simulink model "GTSim_RQ"  (Simulink 7.8)
settings: Solver=ode45  StartTime=0.0  StopTime=3000  RelTol=1e-3
undefined symbols (not defined in the file or in its folder): des_subsystemblock, des_subsysteminport, des_subsystemoutport, des_subsystemsupportblock, MARGIN
libraries: simeventsattributes2 x20, simeventssink1 x17, simeventsrouting1 x15, simeventsgenerators1 x12, simeventstiming1 x4, simeventsqueue1 x1, simeventstranslate1 x1, simeventsserver1 x1
settings Model: Creator=msemamit  LastModifiedBy=msemamit
settings DebuggingCC: FcnCallInpInsideContextMsg=Use local settings
settings SFSimCC: SimParseCustomCode=off
settings SimEventsCC: propDiagAttribOutput=1  propDiagFcnCallOutput=1  propDiagStatOutput=0

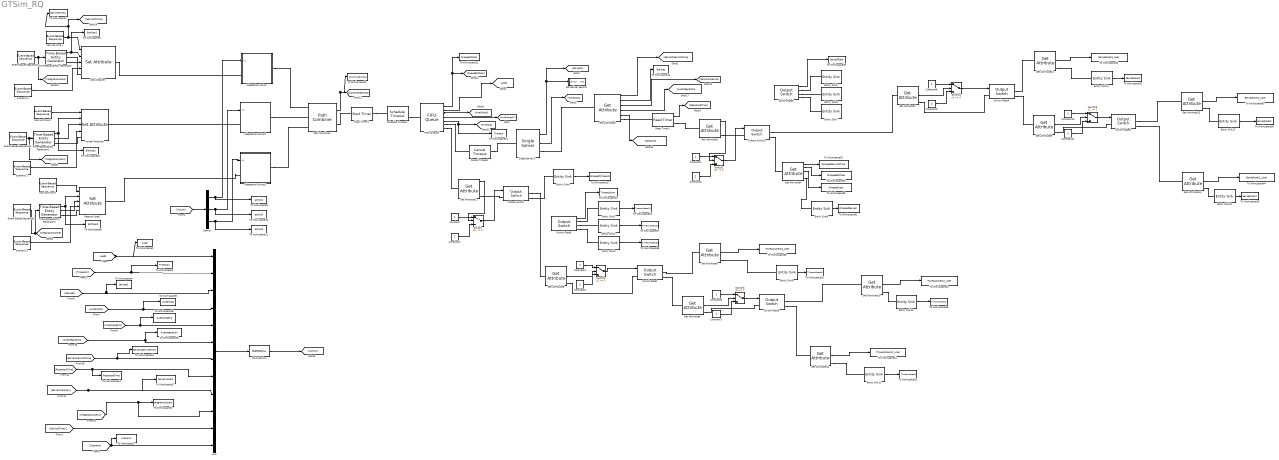
== system GTSim_RQ ==
  Adaptation Action : Subsystem
  Adaptation Action1 : Subsystem
  Adaptation Action2 : Subsystem
  Cancel Timeout : simeventstiming1/Cancel Timeout  Priority=0  TimeoutTag=TO1  TimeoutModeOption=Continue  TimeoutCancelledOption=Error  StatNumberDeparted=Off  StatTimeoutNumberDeparted=Off  StatResidualTimeout=Off  StatAverageResidualTimeout=Off
  Constant{,2,4,6,8,10} (6 alike) : Constant  OutDataTypeStr=double
  Constant{1,3,5,7,9,11} (6 alike) : Constant  Value=2  OutDataTypeStr=double
  Demux : Demux  Outputs=3
  DoS Attacker : simeventsattributes2/Set Attribute  Priority=1  AttributeFrom=Signal port|Signal port|Dialog|Signal port|Signal port  AttributeName=ServiceTime|Entities|User|AveIntegration|Scenario  AttributeTreatAsVector=1|1|1|1|1  AttributeValue=1|1|1|1|1  AttributeCreate=on  StatNumberDeparted=Off  EvaluatedAttributeValue={[];[];1;[];[]}
  Entity Sink{1..14} (14 alike) : simeventssink1/Entity Sink  Priority=1  AvailableForArrivals=on  StatNumberArrived=On
  Event-Based Sequence : simeventsgenerators1/Signal Generators/Event-Based Sequence  VectorOutputValues=user1  FormOutputOpt=Setting to infinity  IsProcessed=on  isConnected=1
  Event-Based Sequence1 : simeventsgenerators1/Signal Generators/Event-Based Sequence  VectorOutputValues=user2  FormOutputOpt=Setting to infinity  IsProcessed=on  isConnected=1
  Event-Based Sequence2 : simeventsgenerators1/Signal Generators/Event-Based Sequence  VectorOutputValues=user3  FormOutputOpt=Setting to infinity  IsProcessed=on  isConnected=1
  FIFO Queue7 : simeventsqueue1/FIFO Queue  Priority=1  Capacity=5000  EnableTOPort=on  StatNumberDeparted=On  StatNumberInBlock=On  StatPendingEntity=Off  StatAverageWait=On  StatAverageQueueLength=On  StatNumberTimedout=On
  Get Attribute{1,3..14} (13 alike) : simeventsattributes2/Get Attribute  Priority=1  AttributeName=ServiceTime|Entities|User|AveIntegration  AttributeMissing=Error|Error|Error|Error  AttributeDefaultValue=1|1|1|1  AttributeSendTiming=After entity departure|After entity departure|After entity departure|After entity departure  AttributeTreatAsVector=1|1|1|1  StatNumberDeparted=Off  EvaluatedDefaultAttributeValue={[];[];[];[]}
  Get Attribute2 : simeventsattributes2/Get Attribute  Priority=1  AttributeName=ServiceTime|Entities|User|AveIntegration|Scenario  AttributeMissing=Error|Error|Error|Error|Error  AttributeDefaultValue=1|1|1|1|1  AttributeSendTiming=After entity departure|After entity departure|After entity departure|After entity departure|After entity departure  AttributeTreatAsVector=1|1|1|1|1  StatNumberDeparted=Off  EvaluatedDefaultAttributeValue={[];[];[];[];[]}
  Insider Attacker : simeventsattributes2/Set Attribute  Priority=1  AttributeFrom=Signal port|Signal port|Dialog|Signal port|Signal port  AttributeName=ServiceTime|Entities|User|AveIntegration|Scenario  AttributeTreatAsVector=1|1|1|1|1  AttributeValue=1|1|2|1|1  AttributeCreate=on  StatNumberDeparted=Off  EvaluatedAttributeValue={[];[];2;[];[]}
  MATLAB Fcn : MATLABFcn  MATLABFcn=MARGIN(u)
  Mux : Mux  Inputs=12
  Output Switch : simeventsrouting1/Output Switch  Priority=1  NumberOutputPorts=2  SwitchingCriterion=From signal port p  InitialSeed=34567  AttributeName=Attribute1  InitialConditionsOpt=off  InitialConditions=1  EntityBufferOpt=on  SpecifyEventPriority=off  PriorityOutputSwitchSelectPort=4100  TimeoutPortOpt=off  StatNumberDeparted=On  StatNumberTimedOut=Off  StatPendingEntity=Off  StatLastDeparturePort=Off  EvaluatedNumPorts=2
  Output Switch1 : simeventsrouting1/Output Switch  Priority=1  NumberOutputPorts=2  SwitchingCriterion=From signal port p  InitialSeed=34567  AttributeName=Attribute1  InitialConditionsOpt=off  InitialConditions=1  EntityBufferOpt=on  SpecifyEventPriority=off  PriorityOutputSwitchSelectPort=4100  TimeoutPortOpt=off  StatNumberDeparted=On  StatNumberTimedOut=Off  StatPendingEntity=Off  StatLastDeparturePort=Off  EvaluatedNumPorts=2
  Path Combiner : simeventsrouting1/Path Combiner  Priority=1  NumberInputPorts=3  InputPortPrecedence=Round robin  InitialSeed=45675  SpecifyEventPriority=off  PriorityPathCombinerPortPrecedenceSelection=4100  StatNumberDeparted=On  StatLastArrivalPort=Off  EvaluatedNumPorts=3
  Read Timer1 : simeventstiming1/Read Timer  Priority=0  TimerTag=T2  TimerModeOption=Error  TimerStop=off  StatNumberDeparted=Off  StatTimerNumberDeparted=Off  StatTimeElapsed=On  StatAverageTimeElapsed=Off
  Regular User1 : simeventsattributes2/Set Attribute  Priority=1  AttributeFrom=Signal port|Signal port|Dialog|Signal port|Signal port  AttributeName=ServiceTime|Entities|User|AveIntegration|Scenario  AttributeTreatAsVector=1|1|1|1|1  AttributeValue=1|1|3|1|1  AttributeCreate=on  StatNumberDeparted=Off  EvaluatedAttributeValue={[];[];3;[];[]}
  Schedule Timeout : simeventstiming1/Schedule Timeout  Priority=0  TimeoutTag=TO1  TimeoutIntervalFrom=Dialog  TimeoutInterval=3000  AttributeName=TimeoutAttribute  PriorityTimeout=1700  TimeoutScheduledOption=Error  TimeoutNoDestination=Error  StatNumberDeparted=On
  Served per Second : Subsystem  LoadFcn=des_subsystemblock(gcb, 'load');  InitFcn=des_subsystemblock(gcb, 'init');  StartFcn=des_subsystemblock(gcb, 'start');  StopFcn=des_subsystemblock(gcb, 'stop');
      settings: CopyFcn=des_subsystemblock(gcb, 'copy');  DeleteFcn=des_subsystemblock(gcb, 'delete');  UndoDeleteFcn=des_subsystemblock(gcb, 'undodelete');  ModelCloseFcn=des_subsystemblock(gcb, 'modelclose');  PreSaveFcn=des_subsystemblock(gcb, 'presave');  NameChangeFcn=des_subsystemblock(gcb, 'namechange');  OpenFcn=des_subsystemblock(gcb, 'open');  ParentCloseFcn=des_subsystemblock(gcb, 'parentclose');  ErrorFcn=des_subsystemerror
      mask Type: Discrete Event Subsystem
      mask Help: helpview(simeventsbhelp);
  Single Server 1 : simeventsserver1/Single Server  Priority=1  ServiceTimeFrom=Attribute  ServiceTime=1  AttributeName=ServiceTime  PriorityServiceCompletion=500  PermitPreemption=off  SortingAttributeName=PriorityAttributeName  SortingDirection=Ascending  WriteToAttribute=off  ResidualAttributeName=ResidualServiceTime  CreateAttribute=on  EnableTOPort=off  StatNumberDeparted=On  StatNumberInBlock=Off  StatNumberPreempted=Off  StatPendingEntity=Off  StatAverageWait=Off  StatUtilization=Off  StatNumberTimedout=On
  Start Timer1 : simeventstiming1/Start Timer  Priority=0  TimerTag=T2  TimerStartedOption=Warn and continue  StatNumberDeparted=Off
  Switch : Switch  Criteria=u2 ~= 0  ZeroCross=off
  Switch Gate{1,3..4,6} (4 alike) : simeventsrouting1/Output Switch  Priority=1  NumberOutputPorts=2  SwitchingCriterion=From signal port p  InitialSeed=34567  AttributeName=User  InitialConditionsOpt=off  InitialConditions=1  EntityBufferOpt=on  SpecifyEventPriority=off  PriorityOutputSwitchSelectPort=4100  TimeoutPortOpt=off  StatNumberDeparted=On  StatNumberTimedOut=Off  StatPendingEntity=Off  StatLastDeparturePort=Off  EvaluatedNumPorts=2
  Switch Gate2 : simeventsrouting1/Output Switch  Priority=1  NumberOutputPorts=3  SwitchingCriterion=From attribute  InitialSeed=34567  AttributeName=User  InitialConditionsOpt=off  InitialConditions=1  EntityBufferOpt=off  SpecifyEventPriority=off  PriorityOutputSwitchSelectPort=4100  TimeoutPortOpt=off  StatNumberDeparted=On  StatNumberTimedOut=Off  StatPendingEntity=Off  StatLastDeparturePort=Off  EvaluatedNumPorts=3
  Switch Gate5 : simeventsrouting1/Output Switch  Priority=1  NumberOutputPorts=3  SwitchingCriterion=From attribute  InitialSeed=34567  AttributeName=User  InitialConditionsOpt=off  InitialConditions=1  EntityBufferOpt=off  SpecifyEventPriority=off  PriorityOutputSwitchSelectPort=4100  TimeoutPortOpt=off  StatNumberDeparted=On  StatNumberTimedOut=Off  StatPendingEntity=Off  StatLastDeparturePort=Off  EvaluatedNumPorts=3
  Switch1 : Switch  Criteria=u2 ~= 0  ZeroCross=off
  Switch2 : Switch  Threshold=3  ZeroCross=off
  Switch3 : Switch  Threshold=2  ZeroCross=off
  Switch4 : Switch  Threshold=3  RndMeth=Ceiling  ZeroCross=off
  Switch5 : Switch  Threshold=2  RndMeth=Ceiling  ZeroCross=off
  Time-Based Entity Generator : simeventsgenerators1/Entity Generators/Time-Based Entity Generator  Priority=1  GenerateEntitiesUpon=Intergeneration time from port t  Distribution=Constant  Minimum=50  Maximum=100  Mean=15  InitialSeed=12345  Period=5  PriorityEntityGeneration=300  GenerateEntityAtSimulationStart=on  ResponseWhenBlocked=Error  ResponseWhenUnblocked=Immediate restart  EntityType=Blank  StatNumberDeparted=On  StatPendingEntity=Off  StatAverageIntergenerationTime=On
  Time-Based Entity Generator1 : simeventsgenerators1/Entity Generators/Time-Based Entity Generator  Priority=1  GenerateEntitiesUpon=Intergeneration time from port t  Distribution=Constant  Minimum=10  Maximum=100  Mean=10  InitialSeed=12345  Period=50  PriorityEntityGeneration=300  GenerateEntityAtSimulationStart=on  ResponseWhenBlocked=Error  ResponseWhenUnblocked=Immediate restart  EntityType=Blank  StatNumberDeparted=On  StatPendingEntity=Off  StatAverageIntergenerationTime=On
  Time-Based Entity Generator2 : simeventsgenerators1/Entity Generators/Time-Based Entity Generator  Priority=1  GenerateEntitiesUpon=Intergeneration time from port t  Distribution=Constant  Minimum=10  Maximum=100  Mean=10  InitialSeed=12345  Period=50  PriorityEntityGeneration=300  GenerateEntityAtSimulationStart=on  ResponseWhenBlocked=Error  ResponseWhenUnblocked=Immediate restart  EntityType=Blank  StatNumberDeparted=On  StatPendingEntity=Off  StatAverageIntergenerationTime=On
  To Workspace1 : ToWorkspace  VariableName=ServiceTime1  SampleTime=-1  SaveFormat=Array
  To Workspace10 : ToWorkspace  VariableName=action2  SampleTime=-1  SaveFormat=Array
  To Workspace11 : ToWorkspace  VariableName=action3  SampleTime=-1  SaveFormat=Array
  To Workspace12 : ToWorkspace  VariableName=ResponseTime  SampleTime=-1  SaveFormat=Array
  To Workspace13 : ToWorkspace  VariableName=Timeout  SampleTime=-1  SaveFormat=Array
  To Workspace14 : ToWorkspace  VariableName=Entities  SampleTime=-1  SaveFormat=Array
  To Workspace15 : ToWorkspace  VariableName=Server1ServiceTime  SampleTime=-1  SaveFormat=Array
  To Workspace16 : ToWorkspace  VariableName=AveQLength1  SampleTime=-1  SaveFormat=Array
  To Workspace17 : ToWorkspace  VariableName=Server1Users  SampleTime=-1  SaveFormat=Array
  To Workspace18 : ToWorkspace  VariableName=AveIntegration  SampleTime=-1  SaveFormat=Array
  To Workspace19 : ToWorkspace  VariableName=Entities2  SampleTime=-1  SaveFormat=Array
  To Workspace2 : ToWorkspace  VariableName=Load  SampleTime=-1  SaveFormat=Array
  To Workspace20 : ToWorkspace  VariableName=IntegrationUser1  SampleTime=-1  SaveFormat=Array
  To Workspace21 : ToWorkspace  VariableName=QueueEntities  SampleTime=-1  SaveFormat=Array
  To Workspace22 : ToWorkspace  VariableName=CombinerEntities  SampleTime=-1  SaveFormat=Array
  To Workspace23 : ToWorkspace  VariableName=TimeoutUsers11  SampleTime=-1  SaveFormat=Array
  To Workspace24 : ToWorkspace  VariableName=TimeoutNum  SampleTime=-1  SaveFormat=Array
  To Workspace25 : ToWorkspace  VariableName=TimeoutUsers1  SampleTime=-1  SaveFormat=Array
  To Workspace26 : ToWorkspace  VariableName=TimeoutUsers3  SampleTime=-1  SaveFormat=Array
  To Workspace27 : ToWorkspace  VariableName=DroppedTimeouts  SampleTime=-1  SaveFormat=Array
  To Workspace28 : ToWorkspace  VariableName=ServedUser1  SampleTime=-1  SaveFormat=Array
  To Workspace29 : ToWorkspace  VariableName=ServedTotal  SampleTime=-1  SaveFormat=Array
  To Workspace3 : ToWorkspace  VariableName=Timeout1  SampleTime=-1  SaveFormat=Array
  To Workspace30 : ToWorkspace  VariableName=ServedUser2  SampleTime=-1  SaveFormat=Array
  To Workspace31 : ToWorkspace  VariableName=ServedUser3  SampleTime=-1  SaveFormat=Array
  To Workspace32 : ToWorkspace  VariableName=DroppedServed  SampleTime=-1  SaveFormat=Array
  To Workspace33 : ToWorkspace  VariableName=DroppedServiceTime  SampleTime=-1  SaveFormat=Array
  To Workspace34 : ToWorkspace  VariableName=DroppedEntities  SampleTime=-1  SaveFormat=Array
  To Workspace35 : ToWorkspace  VariableName=DroppedUser  SampleTime=-1  SaveFormat=Array
  To Workspace36 : ToWorkspace  VariableName=TimeoutUsers2  SampleTime=-1  SaveFormat=Array
  To Workspace37 : ToWorkspace  VariableName=TimeoutUsers22  SampleTime=-1  SaveFormat=Array
  To Workspace38 : ToWorkspace  VariableName=TimeoutUsers33  SampleTime=-1  SaveFormat=Array
  To Workspace39 : ToWorkspace  VariableName=TimeoutUsers3_User  SampleTime=-1  SaveFormat=Array
  To Workspace4 : ToWorkspace  VariableName=Served1  SampleTime=-1  SaveFormat=Array
  To Workspace40 : ToWorkspace  VariableName=TimeoutUsers2_User  SampleTime=-1  SaveFormat=Array
  To Workspace41 : ToWorkspace  VariableName=TimeoutUsers1_User  SampleTime=-1  SaveFormat=Array
  To Workspace42 : ToWorkspace  VariableName=ServedUser3_User  SampleTime=-1  SaveFormat=Array
  To Workspace43 : ToWorkspace  VariableName=ServedUser2_User  SampleTime=-1  SaveFormat=Array
  To Workspace44 : ToWorkspace  VariableName=ServedUser1_User  SampleTime=-1  SaveFormat=Array
  To Workspace5 : ToWorkspace  VariableName=Entities1  SampleTime=-1  SaveFormat=Array
  To Workspace6 : ToWorkspace  VariableName=Entities3  SampleTime=-1  SaveFormat=Array
  To Workspace7 : ToWorkspace  VariableName=scenario  SampleTime=-1  SaveFormat=Array
  To Workspace8 : ToWorkspace  VariableName=AveQWait  SampleTime=-1  SaveFormat=Array
  To Workspace9 : ToWorkspace  VariableName=action1  SampleTime=-1  SaveFormat=Array
  scenario 1 : simeventsgenerators1/Signal Generators/Event-Based Sequence  VectorOutputValues=scenario1  FormOutputOpt=Setting to zero  IsProcessed=on  isConnected=1
  scenario 2 : simeventsgenerators1/Signal Generators/Event-Based Sequence  VectorOutputValues=scenario2  FormOutputOpt=Setting to zero  IsProcessed=on  isConnected=1
  scenario 3 : simeventsgenerators1/Signal Generators/Event-Based Sequence  VectorOutputValues=scenario3  FormOutputOpt=Setting to zero  IsProcessed=on  isConnected=1
  service time 1 : simeventsgenerators1/Signal Generators/Event-Based Sequence  VectorOutputValues=st1  FormOutputOpt=Cyclic repetition  IsProcessed=on  isConnected=1
  service time 2 : simeventsgenerators1/Signal Generators/Event-Based Sequence  VectorOutputValues=st2  FormOutputOpt=Cyclic repetition  IsProcessed=on  isConnected=1
  service time 3 : simeventsgenerators1/Signal Generators/Event-Based Sequence  VectorOutputValues=st3  FormOutputOpt=Cyclic repetition  IsProcessed=on  isConnected=1
  tag scope: Load1=global
  wires:
  Single Server 1/1 -> [Served1], Served per Second/1(served)
  Single Server 1/2 -> [Timeout1]
  Time-Based Entity Generator/1 -> To Workspace5/1, DoS Attacker/2
  Event-Based Sequence/1 -> Time-Based Entity Generator/1, [IntegrationUser1]
  [Server1Usersss] -> To Workspace17/1, Mux/9
  [Server1ServiceTime] -> To Workspace15/1, Mux/7
  [AveIntegration] -> Mux/6, To Workspace18/1
  [ResponseTime] -> To Workspace12/1, Mux/8
  Mux/1 -> MATLAB Fcn/1
  [AveQWait] -> Mux/4, To Workspace8/1
  [Served1] -> Mux/3, To Workspace4/1
  MATLAB Fcn/1 -> [Action]
  [Timeout1] -> Mux/2, To Workspace3/1
  [Load1] -> Mux/1, To Workspace2/1
  [Scenario] -> Mux/12, To Workspace7/1
  [IntegrationUser1] -> Mux/10, To Workspace20/1
  [ServiceTime1] -> Mux/11
  [AveQLength1] -> Mux/5, To Workspace16/1
  FIFO Queue7/4 -> [AveQLength1]
  FIFO Queue7/3 -> [AveQWait]
  FIFO Queue7/2 -> [Load1]
  Read Timer1/1 -> [ResponseTime]
  [Action] -> Demux/1
  Demux/1 -> Adaptation Action/1(In1), To Workspace9/1
  Time-Based Entity Generator2/1 -> To Workspace19/1, Insider Attacker/2
  Time-Based Entity Generator2/2 -> Insider Attacker/3
  Event-Based Sequence1/1 -> Time-Based Entity Generator2/1, [IntegrationUser2]
  Time-Based Entity Generator1/1 -> To Workspace6/1, Regular User1/2
  Event-Based Sequence2/1 -> [IntegrationUser3], Time-Based Entity Generator1/1
  Time-Based Entity Generator1/2 -> Regular User1/3
  service time 2/1 -> Insider Attacker/1
  service time 3/1 -> Regular User1/1
  Demux/2 -> To Workspace10/1, Adaptation Action1/1(In1)
  Demux/3 -> To Workspace11/1, Adaptation Action2/1(In1)
  FIFO Queue7/5 -> [Timeout], To Workspace13/1
  FIFO Queue7/1 -> [QueueEntities], To Workspace21/1
  Path Combiner/1 -> [CombinerEntities], To Workspace22/1
  Time-Based Entity Generator/2 -> DoS Attacker/3
  service time 1/1 -> [ServiceTime1], To Workspace1/1, DoS Attacker/1
  Switch Gate5/1 -> To Workspace24/1
  Constant/1 -> Switch/1
  Constant1/1 -> Switch/3
  Entity Sink4/1 -> To Workspace27/1
  Get Attribute1/1 -> Switch/2
  Switch/1 -> Output Switch/1
  Switch Gate2/1 -> To Workspace29/1
  Constant2/1 -> Switch1/1
  Constant3/1 -> Switch1/3
  Entity Sink8/1 -> To Workspace32/1
  Get Attribute3/1 -> Switch1/2
  Switch1/1 -> Output Switch1/1
  Get Attribute4/1 -> To Workspace33/1
  Get Attribute4/2 -> To Workspace34/1
  Get Attribute4/3 -> To Workspace35/1
  Constant4/1 -> Switch2/1
  Constant5/1 -> Switch2/3
  Switch2/1 -> Switch Gate1/1
  Constant6/1 -> Switch3/1
  Constant7/1 -> Switch3/3
  Get Attribute6/3 -> Switch3/2
  Switch3/1 -> Switch Gate3/1
  Entity Sink1/1 -> To Workspace23/1
  Entity Sink3/1 -> To Workspace38/1
  Entity Sink2/1 -> To Workspace37/1
  Constant8/1 -> Switch4/1
  Constant9/1 -> Switch4/3
  Constant10/1 -> Switch5/1
  Constant11/1 -> Switch5/3
  Get Attribute8/3 -> Switch5/2
  Switch5/1 -> Switch Gate6/1
  Get Attribute9/3 -> To Workspace39/1
  Get Attribute10/3 -> To Workspace40/1
  Get Attribute11/3 -> To Workspace41/1
  Get Attribute12/3 -> To Workspace42/1
  Get Attribute14/3 -> To Workspace44/1
  Get Attribute13/3 -> To Workspace43/1
  Get Attribute5/3 -> Switch2/2
  Entity Sink11/1 -> To Workspace25/1
  Entity Sink10/1 -> To Workspace36/1
  Entity Sink9/1 -> To Workspace26/1
  Get Attribute7/3 -> Switch4/2
  Entity Sink14/1 -> To Workspace31/1
  Entity Sink12/1 -> To Workspace30/1
  Entity Sink13/1 -> To Workspace28/1
  Switch4/1 -> Switch Gate4/1
  scenario 1/1 -> DoS Attacker/4
  scenario 2/1 -> Insider Attacker/4
  scenario 3/1 -> Regular User1/4
  Get Attribute2/1 -> [Server1ServiceTime]
  Get Attribute2/2 -> To Workspace14/1
  Get Attribute2/3 -> [Server1Usersss]
  Get Attribute2/4 -> [AveIntegration]
  Get Attribute2/5 -> [Scenario]
  connections:
  Time-Based Entity Generator/RConn1 -- DoS Attacker/LConn1
  Get Attribute2/RConn1 -- Read Timer1/LConn1
  DoS Attacker/RConn1 -- Adaptation Action/LConn1
  Adaptation Action/RConn1 -- Path Combiner/LConn1
  Regular User1/RConn1 -- Adaptation Action2/LConn1
  Insider Attacker/RConn1 -- Adaptation Action1/LConn1
  Time-Based Entity Generator2/RConn1 -- Insider Attacker/LConn1
  Time-Based Entity Generator1/RConn1 -- Regular User1/LConn1
  Adaptation Action1/RConn1 -- Path Combiner/LConn2
  Adaptation Action2/RConn1 -- Path Combiner/LConn3
  Path Combiner/RConn1 -- Start Timer1/LConn1
  Start Timer1/RConn1 -- Schedule Timeout/LConn1
  Schedule Timeout/RConn1 -- FIFO Queue7/LConn1
  Single Server 1/RConn1 -- Get Attribute2/LConn1
  Cancel Timeout/RConn1 -- Single Server 1/LConn1
  FIFO Queue7/RConn1 -- Cancel Timeout/LConn1
  Switch Gate5/RConn1 -- Entity Sink1/LConn1
  Switch Gate5/RConn2 -- Entity Sink2/LConn1
  Switch Gate5/RConn3 -- Entity Sink3/LConn1
  FIFO Queue7/RConn2 -- Get Attribute1/LConn1
  Output Switch/RConn2 -- Entity Sink4/LConn1
  Get Attribute1/RConn1 -- Output Switch/LConn1
  Switch Gate2/RConn3 -- Entity Sink7/LConn1
  Switch Gate2/RConn2 -- Entity Sink6/LConn1
  Switch Gate2/RConn1 -- Entity Sink5/LConn1
  Get Attribute3/RConn1 -- Output Switch1/LConn1
  Read Timer1/RConn1 -- Get Attribute3/LConn1
  Output Switch1/RConn2 -- Get Attribute4/LConn1
  Get Attribute4/RConn1 -- Entity Sink8/LConn1
  Switch Gate1/RConn2 -- Get Attribute6/LConn1
  Output Switch/RConn1 -- Get Attribute5/LConn1
  Get Attribute6/RConn1 -- Switch Gate3/LConn1
  Get Attribute8/RConn1 -- Switch Gate6/LConn1
  Switch Gate4/RConn2 -- Get Attribute8/LConn1
  Output Switch1/RConn1 -- Get Attribute7/LConn1
  Switch Gate1/RConn1 -- Get Attribute9/LConn1
  Get Attribute9/RConn1 -- Entity Sink9/LConn1
  Switch Gate3/RConn1 -- Get Attribute10/LConn1
  Get Attribute10/RConn1 -- Entity Sink10/LConn1
  Switch Gate3/RConn2 -- Get Attribute11/LConn1
  Get Attribute11/RConn1 -- Entity Sink11/LConn1
  Switch Gate4/RConn1 -- Get Attribute12/LConn1
  Get Attribute12/RConn1 -- Entity Sink14/LConn1
  Switch Gate6/RConn1 -- Get Attribute13/LConn1
  Get Attribute13/RConn1 -- Entity Sink12/LConn1
  Switch Gate6/RConn2 -- Get Attribute14/LConn1
  Get Attribute14/RConn1 -- Entity Sink13/LConn1
  Get Attribute5/RConn1 -- Switch Gate1/LConn1
  Get Attribute7/RConn1 -- Switch Gate4/LConn1

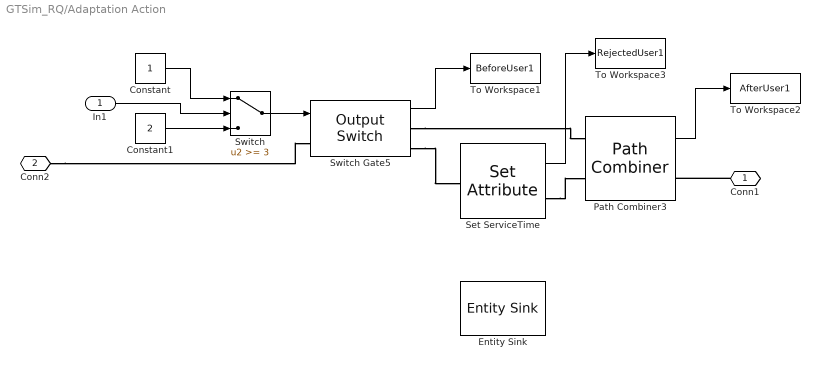
== system GTSim_RQ/Adaptation Action ==
  In1 : Inport
  Constant : Constant
  Constant1 : Constant  Value=2
  Entity Sink : simeventssink1/Entity Sink  Priority=1  AvailableForArrivals=on  StatNumberArrived=On
  Path Combiner3 : simeventsrouting1/Path Combiner  Priority=1  NumberInputPorts=2  InputPortPrecedence=IN1 port  InitialSeed=45675  SpecifyEventPriority=off  PriorityPathCombinerPortPrecedenceSelection=4100  StatNumberDeparted=On  StatLastArrivalPort=Off  EvaluatedNumPorts=2
  Set ServiceTime : simeventsattributes2/Set Attribute  Priority=1  AttributeFrom=Dialog  AttributeName=ServiceTime  AttributeTreatAsVector=1  AttributeValue=0  AttributeCreate=on  StatNumberDeparted=On  EvaluatedAttributeValue={0}
  Switch : Switch  Threshold=3
  Switch Gate5 : simeventsrouting1/Output Switch  Priority=1  NumberOutputPorts=2  SwitchingCriterion=From signal port p  InitialSeed=34567  AttributeName=User  InitialConditionsOpt=off  InitialConditions=1  EntityBufferOpt=off  SpecifyEventPriority=off  PriorityOutputSwitchSelectPort=4100  TimeoutPortOpt=off  StatNumberDeparted=On  StatNumberTimedOut=Off  StatPendingEntity=Off  StatLastDeparturePort=Off  EvaluatedNumPorts=2
  To Workspace1 : ToWorkspace  VariableName=BeforeUser1  SampleTime=-1  SaveFormat=Array
  To Workspace2 : ToWorkspace  VariableName=AfterUser1  SampleTime=-1  SaveFormat=Array
  To Workspace3 : ToWorkspace  VariableName=RejectedUser1  SampleTime=-1  SaveFormat=Array
  Conn1 : PMIOPort  Port=1  Side=Right
  Conn2 : PMIOPort  Port=2  Side=Left
  wires:
  Switch Gate5/1 -> To Workspace1/1
  Set ServiceTime/1 -> To Workspace3/1
  Path Combiner3/1 -> To Workspace2/1
  Switch/1 -> Switch Gate5/1
  Constant/1 -> Switch/1
  Constant1/1 -> Switch/3
  In1/1 -> Switch/2
  connections:
  Switch Gate5/RConn1 -- Path Combiner3/LConn1
  Conn2/RConn1 -- Switch Gate5/LConn1
  Conn1/RConn1 -- Path Combiner3/RConn1
  Set ServiceTime/RConn1 -- Path Combiner3/LConn2
  Switch Gate5/RConn2 -- Set ServiceTime/LConn1

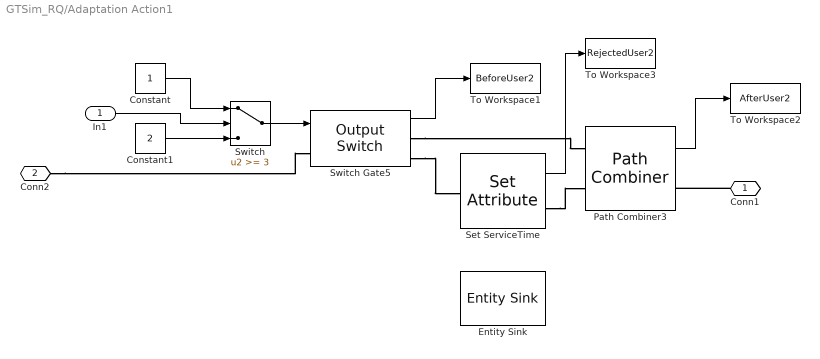
== system GTSim_RQ/Adaptation Action1 ==
  In1 : Inport
  Constant : Constant
  Constant1 : Constant  Value=2
  Entity Sink : simeventssink1/Entity Sink  Priority=1  AvailableForArrivals=on  StatNumberArrived=Off
  Path Combiner3 : simeventsrouting1/Path Combiner  Priority=1  NumberInputPorts=2  InputPortPrecedence=IN1 port  InitialSeed=45675  SpecifyEventPriority=off  PriorityPathCombinerPortPrecedenceSelection=4100  StatNumberDeparted=On  StatLastArrivalPort=Off  EvaluatedNumPorts=2
  Set ServiceTime : simeventsattributes2/Set Attribute  Priority=1  AttributeFrom=Dialog  AttributeName=ServiceTime  AttributeTreatAsVector=1  AttributeValue=0  AttributeCreate=on  StatNumberDeparted=On  EvaluatedAttributeValue={0}
  Switch : Switch  Threshold=3
  Switch Gate5 : simeventsrouting1/Output Switch  Priority=1  NumberOutputPorts=2  SwitchingCriterion=From signal port p  InitialSeed=34567  AttributeName=User  InitialConditionsOpt=off  InitialConditions=1  EntityBufferOpt=off  SpecifyEventPriority=off  PriorityOutputSwitchSelectPort=4100  TimeoutPortOpt=off  StatNumberDeparted=On  StatNumberTimedOut=Off  StatPendingEntity=Off  StatLastDeparturePort=Off  EvaluatedNumPorts=2
  To Workspace1 : ToWorkspace  VariableName=BeforeUser2  SampleTime=-1  SaveFormat=Array
  To Workspace2 : ToWorkspace  VariableName=AfterUser2  SampleTime=-1  SaveFormat=Array
  To Workspace3 : ToWorkspace  VariableName=RejectedUser2  SampleTime=-1  SaveFormat=Array
  Conn1 : PMIOPort  Port=1  Side=Right
  Conn2 : PMIOPort  Port=2  Side=Left
  wires:
  Switch/1 -> Switch Gate5/1
  Constant/1 -> Switch/1
  Constant1/1 -> Switch/3
  In1/1 -> Switch/2
  Path Combiner3/1 -> To Workspace2/1
  Switch Gate5/1 -> To Workspace1/1
  Set ServiceTime/1 -> To Workspace3/1
  connections:
  Switch Gate5/RConn1 -- Path Combiner3/LConn1
  Conn2/RConn1 -- Switch Gate5/LConn1
  Conn1/RConn1 -- Path Combiner3/RConn1
  Set ServiceTime/RConn1 -- Path Combiner3/LConn2
  Switch Gate5/RConn2 -- Set ServiceTime/LConn1

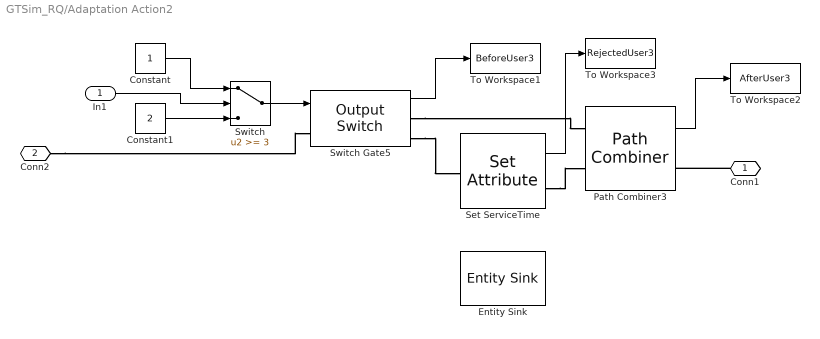
== system GTSim_RQ/Adaptation Action2 ==
  In1 : Inport
  Constant : Constant
  Constant1 : Constant  Value=2
  Entity Sink : simeventssink1/Entity Sink  Priority=1  AvailableForArrivals=on  StatNumberArrived=Off
  Path Combiner3 : simeventsrouting1/Path Combiner  Priority=1  NumberInputPorts=2  InputPortPrecedence=IN1 port  InitialSeed=45675  SpecifyEventPriority=off  PriorityPathCombinerPortPrecedenceSelection=4100  StatNumberDeparted=On  StatLastArrivalPort=Off  EvaluatedNumPorts=2
  Set ServiceTime : simeventsattributes2/Set Attribute  Priority=1  AttributeFrom=Dialog  AttributeName=ServiceTime  AttributeTreatAsVector=1  AttributeValue=0  AttributeCreate=on  StatNumberDeparted=On  EvaluatedAttributeValue={0}
  Switch : Switch  Threshold=3
  Switch Gate5 : simeventsrouting1/Output Switch  Priority=1  NumberOutputPorts=2  SwitchingCriterion=From signal port p  InitialSeed=34567  AttributeName=User  InitialConditionsOpt=off  InitialConditions=1  EntityBufferOpt=off  SpecifyEventPriority=off  PriorityOutputSwitchSelectPort=4100  TimeoutPortOpt=off  StatNumberDeparted=On  StatNumberTimedOut=Off  StatPendingEntity=Off  StatLastDeparturePort=Off  EvaluatedNumPorts=2
  To Workspace1 : ToWorkspace  VariableName=BeforeUser3  SampleTime=-1  SaveFormat=Array
  To Workspace2 : ToWorkspace  VariableName=AfterUser3  SampleTime=-1  SaveFormat=Array
  To Workspace3 : ToWorkspace  VariableName=RejectedUser3  SampleTime=-1  SaveFormat=Array
  Conn1 : PMIOPort  Port=1  Side=Right
  Conn2 : PMIOPort  Port=2  Side=Left
  wires:
  Switch/1 -> Switch Gate5/1
  Constant/1 -> Switch/1
  Constant1/1 -> Switch/3
  In1/1 -> Switch/2
  Path Combiner3/1 -> To Workspace2/1
  Switch Gate5/1 -> To Workspace1/1
  Set ServiceTime/1 -> To Workspace3/1
  connections:
  Switch Gate5/RConn1 -- Path Combiner3/LConn1
  Conn2/RConn1 -- Switch Gate5/LConn1
  Conn1/RConn1 -- Path Combiner3/RConn1
  Set ServiceTime/RConn1 -- Path Combiner3/LConn2
  Switch Gate5/RConn2 -- Set ServiceTime/LConn1

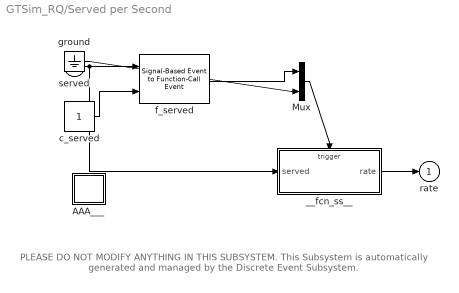
== system GTSim_RQ/Served per Second ==
  note: PLEASE DO NOT MODIFY ANYTHING IN THIS SUBSYSTEM.
      | This Subsystem is automatically generated and
      | managed by the Discrete Event Subsystem.
  served : Inport  OutDataTypeStr=double
  AAA___ : Subsystem  LoadFcn=des_subsystemsupportblock(gcb, 'load');  InitFcn=des_subsystemsupportblock(gcb, 'init');  StartFcn=des_subsystemsupportblock(gcb, 'start');  StopFcn=des_subsystemsupportblock(gcb, 'stop');
      settings: CopyFcn=des_subsystemsupportblock(gcb, 'copy');  DeleteFcn=des_subsystemsupportblock(gcb, 'delete');  UndoDeleteFcn=des_subsystemsupportblock(gcb, 'undodelete');  ModelCloseFcn=des_subsystemsupportblock(gcb, 'modelclose');  PreSaveFcn=des_subsystemsupportblock(gcb, 'presave');  NameChangeFcn=des_subsystemsupportblock(gcb, 'namechange');  OpenFcn=des_subsystemsupportblock(gcb, 'open');  ParentCloseFcn=des_subsystemsupportblock(gcb, 'parentclose');
  Mux : Mux  Inputs=2
  __fcn_ss__ : Subsystem  TreatAsAtomicUnit=on
      settings: PropExecContextOutsideSubsystem=on
  c_served : Constant
  f_served : simeventstranslate1/Signal-Based Event to Function-Call Event  Priority=1  GenerateFunctionCallUpon=Sample time hit from port ts  SignalEdgeOption=Rising  EnableE1Port=on  EnableF2Port=off  EnableE2Port=off  SpecifyEventPriority=off  PriorityFunctionCall=20  FunctionCallDelayFrom=Dialog  DelayFunctionCall=0  StatNumberF1Calls=Off  StatNumberF2Calls=Off  MaskBlockType=DESS_EVENT_PORT
  ground : Ground
  rate : Outport
  wires:
  ground/1 -> Mux/2
  Mux/1 -> __fcn_ss__/Trigger
  c_served/1 -> f_served/2
  f_served/1 -> Mux/1
  __fcn_ss__/1(rate) -> rate/1
  served/1 -> f_served/1, __fcn_ss__/1(served)

== system GTSim_RQ/Served per Second/AAA___ ==

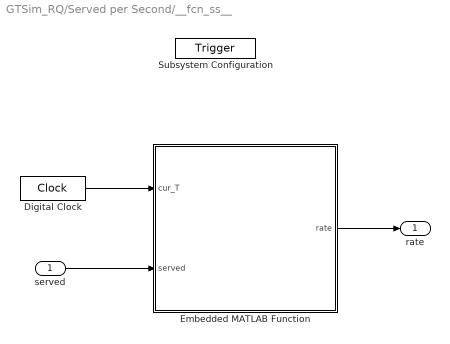
== system GTSim_RQ/Served per Second/__fcn_ss__ ==
  served : Inport  LoadFcn=des_subsysteminport(gcb, 'load');  InitFcn=des_subsysteminport(gcb, 'init');  StartFcn=des_subsysteminport(gcb, 'start');  StopFcn=des_subsysteminport(gcb, 'stop');  mask(Discrete Event Inport){PermitSubsystemEvents=on, TypeOfEvent=Sample time hit, SignalEdgeOption=Rising, SpecifyEventPriority=off, PrioritySubsystemEvent=20}
      mask prompts: PermitSubsystemEvents "Execute subsystem upon signal-based events"; TypeOfEvent "Type of signal-based event:"; SignalEdgeOption "Type of change in signal value:"; SpecifyEventPriority "Specify event priority for executing subsystem"; PrioritySubsystemEvent "Subsystem execution event priority:"
      mask help: Input port for a Discrete Event Subsystem block. This block can conditionally execute the subsystem upon signal-based events that meet specified criteria.
      mask init:
      | des_subsystemmask(gcb, 'init','apply')
      settings: CopyFcn=des_subsysteminport(gcb, 'copy');  ModelCloseFcn=des_subsysteminport(gcb, 'modelclose');  PreSaveFcn=des_subsysteminport(gcb, 'presave');  NameChangeFcn=des_subsysteminport(gcb, 'namechange');  ParentCloseFcn=des_subsysteminport(gcb, 'parentclose');
      mask Help: helpview(simeventsbhelp);
      mask StyleString: checkbox,popup(Change in signal|Trigger|Sample time hit),popup(Rising|Falling|Either),checkbox,edit
      mask CallbackString: des_subsystemmask(gcb, 'cbPermitSubsystemEvents', 'noapply');|des_subsystemmask(gcb,'cbTypeOfEvent','noapply');||des_subsystemmask(gcb, 'cbSpecifyEventPriority', 'noapply');|
  Subsystem Configuration : TriggerPort  TriggerType=function-call
      settings: CopyFcn=des_subsystemconfigblock(gcb, 'copy');
      mask Type: Subsystem Configuration
      mask Description: Configuration for a Discrete Event Subsystem block. Every discrete event subsystem window must contain exactly one copy of this configuration block. Do not delete this block.
      mask Help: helpview(simeventsbhelp);
      mask Display: disp('Do Not Delete');
  Digital Clock : DigitalClock  SampleTime=-1
  Embedded MATLAB Function : MATLAB Function  TreatAsAtomicUnit=on
  rate : Outport  LoadFcn=des_subsystemoutport(gcb, 'load');  InitFcn=des_subsystemoutport(gcb, 'init');  StartFcn=des_subsystemoutport(gcb, 'start');  StopFcn=des_subsystemoutport(gcb, 'stop');
      settings: CopyFcn=des_subsystemoutport(gcb, 'copy');  ModelCloseFcn=des_subsystemoutport(gcb, 'modelclose');  PreSaveFcn=des_subsystemoutport(gcb, 'presave');  NameChangeFcn=des_subsystemoutport(gcb, 'namechange');  ParentCloseFcn=des_subsystemoutport(gcb, 'parentclose');
      mask Type: Discrete Event Outport
      mask Description: Provide an output port for a Discrete Event Subsystem block.
      mask Help: helpview(simeventsbhelp);
  wires:
  Digital Clock/1 -> Embedded MATLAB Function/1(cur_T)
  served/1 -> Embedded MATLAB Function/2(served)
  Embedded MATLAB Function/1(rate) -> rate/1

== matlab function Served per Second/__fcn_ss__/Embedded MATLAB Function ==
  data: cur_T input double; served input double; rate output double
function rate = throughput(cur_T, served)
% THROUGHPUT Compute the rate at which the computer sends data 
% INPUT:
%     cur_T     -- Current simulation time
%     pck_size  -- Size, in bits, of the packet that is successfully
%                  transmitted.
% OUTPUT:
%     rate      -- Current throughput of the computer (in kbps)

%persistent acc_sum;

% Initialize persistent variables in the first iteration.
%if isempty(acc_sum)
%   acc_sum = 0;
%end

% Update the throughput of current computer.
%acc_sum = acc_sum + served;
if cur_T > 10 
    rate = served / (cur_T/10);
else
    rate = 2;
end
